simulink model "Stromregelkreis_old"  (R2024b)
settings: Solver=FixedStepAuto  StartTime=0.0  StopTime=inf  FixedStep=ta  RelTol=1e-3
PostLoadFcn:
  | if any(exist('dsrtsu_mdlpostloadfcn', 'file') ~= 0), dsrtsu_mdlpostloadfcn('Execute', bdroot); end
InitFcn:
  | , if any(exist('rtifpga_mdlclblib', 'file') ~= 0), rtifpga_mdlclblib('Init', bdroot); end,
undefined symbols (not defined in the file or in its folder): ta
libraries: rtilib1104 x20, simulink x4
settings Model: DSRTSU_INTERNAL_RTI_VER=650  DSRTSU_INTERNAL_RTI_TYPE=rti1104  DSRTSU_INTERNAL_RTIFPGA=210  DSRTSU_INTERNAL_RTISTBM_VER=24.2  Creator=115145  LastModifiedBy=217836
settings OptimizationCC: BlockReduction=off  OptimizeBlockIOStorage=off
settings HardwareCC: ProdBitPerPointer=32  ProdBitPerSizeT=32  ProdBitPerPtrDiffT=32  ProdLargestAtomicInteger=Integer  ProdEndianess=BigEndian  ProdWordSize=32  ProdHWDeviceType=Custom Processor->Custom  TargetIntDivRoundTo=Zero  TargetEndianess=BigEndian  TargetHWDeviceType=Custom Processor->Custom
settings SFSimCC: MATLABDynamicMemAlloc=off
settings RTWCC: Description=dSPACE DS1104 Hardware Platform  SystemTargetFile=rti1104.tlc  MakeCommand=make_rti  TemplateMakefile=rti1104.tmf
settings STFCustomTargetCC: ParMdlRefBuildCompliant=on  SystemTargetFile=rti1104.tlc
settings GRTTargetCC: TargetLangStandard=C89/C90 (ANSI)  CompOptLevelCompliant=off  ConcurrentExecutionCompliant=off  CombineOutputUpdateFcns=off  MatFileLogging=off  CPPClassGenCompliant=off  UseToolchainInfoCompliant=off

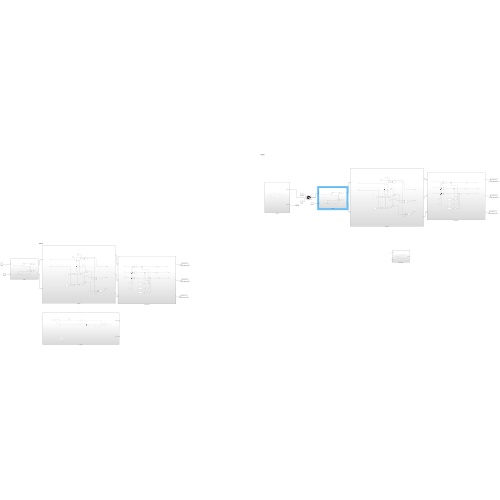
[thumbnail: Simulink's stored preview of the top-level diagram]
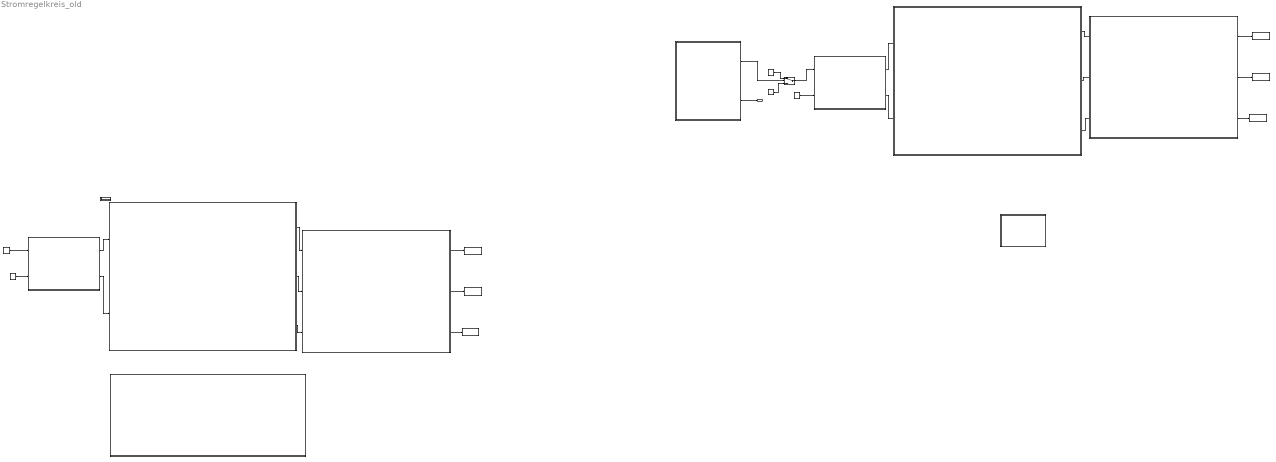
== system Stromregelkreis_old ==
  DS1104SL_DSP_BIT_OUT_C1 : rtilib1104/DS1104 SLAVE DSP/DS1104SL_DSP_BIT_OUT_C0  ChannelNo=1  InitValue=0  TermMode=0  TermValue=0  Reserved1=[]  Reserved2=[]  Reserved3=[]  Reserved=[]  DialogFcn=gui1104sl_dsp_bit_out  UnitName={'DS1104SL_DSP_BIT_OUT_C'}  UnitValues={1}  DSProperties=struct('RTI',struct('Version',uint32(1),'BlockType',struct('isSLSource',uint8(0),'isSLSink',uint8(1),'isHWSource',uint8(0),'isHWSink',uint8(1),'isSetup',uint8(0),'isInline',uint8(1),'isNonInline',uint8(0),'isInterrupt',uint8(0),'isChannelwise',uint8(1)),'IOBoardType','DS1104SLAVE','UnitType','BIT','Identifier','BITOUTCH','DialogType','ML','BlockSet','NONE','SlaveProcessor','F240'))
      settings: SourceProductName=dSPACE RTI1104
  DS1104SL_DSP_BIT_OUT_C2 : rtilib1104/DS1104 SLAVE DSP/DS1104SL_DSP_BIT_OUT_C0  ChannelNo=2  InitValue=0  TermMode=0  TermValue=0  Reserved1=[]  Reserved2=[]  Reserved3=[]  Reserved=[]  DialogFcn=gui1104sl_dsp_bit_out  UnitName={'DS1104SL_DSP_BIT_OUT_C'}  UnitValues={2}  DSProperties=struct('RTI',struct('Version',uint32(1),'BlockType',struct('isSLSource',uint8(0),'isSLSink',uint8(1),'isHWSource',uint8(0),'isHWSink',uint8(1),'isSetup',uint8(0),'isInline',uint8(1),'isNonInline',uint8(0),'isInterrupt',uint8(0),'isChannelwise',uint8(1)),'IOBoardType','DS1104SLAVE','UnitType','BIT','Identifier','BITOUTCH','DialogType','ML','BlockSet','NONE','SlaveProcessor','F240'))
      settings: SourceProductName=dSPACE RTI1104
  DS1104SL_DSP_BIT_OUT_C3 : rtilib1104/DS1104 SLAVE DSP/DS1104SL_DSP_BIT_OUT_C0  ChannelNo=3  InitValue=0  TermMode=0  TermValue=0  Reserved1=[]  Reserved2=[]  Reserved3=[]  Reserved=[]  DialogFcn=gui1104sl_dsp_bit_out  UnitName={'DS1104SL_DSP_BIT_OUT_C'}  UnitValues={ 3 }  DSProperties=struct('RTI',struct('Version',uint32(1),'BlockType',struct('isSLSource',uint8(0),'isSLSink',uint8(1),'isHWSource',uint8(0),'isHWSink',uint8(1),'isSetup',uint8(0),'isInline',uint8(1),'isNonInline',uint8(0),'isInterrupt',uint8(0),'isChannelwise',uint8(1)),'IOBoardType','DS1104SLAVE','UnitType','BIT','Identifier','BITOUTCH','DialogType','ML','BlockSet','NONE','SlaveProcessor','F240'))
      settings: SourceProductName=dSPACE RTI1104
  DS1104SL_DSP_BIT_OUT_C4 : rtilib1104/DS1104 SLAVE DSP/DS1104SL_DSP_BIT_OUT_C0  ChannelNo=4  InitValue=0  TermMode=0  TermValue=0  Reserved1=[]  Reserved2=[]  Reserved3=[]  Reserved=[]  DialogFcn=gui1104sl_dsp_bit_out  UnitName={'DS1104SL_DSP_BIT_OUT_C'}  UnitValues={ 4 }  DSProperties=struct('RTI',struct('Version',uint32(1),'BlockType',struct('isSLSource',uint8(0),'isSLSink',uint8(1),'isHWSource',uint8(0),'isHWSink',uint8(1),'isSetup',uint8(0),'isInline',uint8(1),'isNonInline',uint8(0),'isInterrupt',uint8(0),'isChannelwise',uint8(1)),'IOBoardType','DS1104SLAVE','UnitType','BIT','Identifier','BITOUTCH','DialogType','ML','BlockSet','NONE','SlaveProcessor','F240'))
      settings: SourceProductName=dSPACE RTI1104
  DS1104SL_DSP_BIT_OUT_C5 : rtilib1104/DS1104 SLAVE DSP/DS1104SL_DSP_BIT_OUT_C0  ChannelNo=5  InitValue=0  TermMode=0  TermValue=0  Reserved1=[]  Reserved2=[]  Reserved3=[]  Reserved=[]  DialogFcn=gui1104sl_dsp_bit_out  UnitName={'DS1104SL_DSP_BIT_OUT_C'}  UnitValues={ 5 }  DSProperties=struct('RTI',struct('Version',uint32(1),'BlockType',struct('isSLSource',uint8(0),'isSLSink',uint8(1),'isHWSource',uint8(0),'isHWSink',uint8(1),'isSetup',uint8(0),'isInline',uint8(1),'isNonInline',uint8(0),'isInterrupt',uint8(0),'isChannelwise',uint8(1)),'IOBoardType','DS1104SLAVE','UnitType','BIT','Identifier','BITOUTCH','DialogType','ML','BlockSet','NONE','SlaveProcessor','F240'))
      settings: SourceProductName=dSPACE RTI1104
  DS1104SL_DSP_BIT_OUT_C6 : rtilib1104/DS1104 SLAVE DSP/DS1104SL_DSP_BIT_OUT_C0  ChannelNo=6  InitValue=0  TermMode=0  TermValue=0  Reserved1=[]  Reserved2=[]  Reserved3=[]  Reserved=[]  DialogFcn=gui1104sl_dsp_bit_out  UnitName={'DS1104SL_DSP_BIT_OUT_C'}  UnitValues={6}  DSProperties=struct('RTI',struct('Version',uint32(1),'BlockType',struct('isSLSource',uint8(0),'isSLSink',uint8(1),'isHWSource',uint8(0),'isHWSink',uint8(1),'isSetup',uint8(0),'isInline',uint8(1),'isNonInline',uint8(0),'isInterrupt',uint8(0),'isChannelwise',uint8(1)),'IOBoardType','DS1104SLAVE','UnitType','BIT','Identifier','BITOUTCH','DialogType','ML','BlockSet','NONE','SlaveProcessor','F240'))
      settings: SourceProductName=dSPACE RTI1104
  Iq_soll : Constant  Value=0
  RTI Data : Subsystem  Tag=struct('RTIDataServer',struct('RTIDataServerVs','2','RTIModelDescription','struct(''main'',''Stromregelkreis_old'',''sub'',''Stromregelkreis_old'',''isMp'',0)'))  LoadFcn="if exist('rtidc'), try,  rtidc('DataHostBlockClbLoad', gcbh); catch, disp(['Warning: ''LoadFcn'' for RTI Data block failed: ' lasterr]); end, end,"  mask(RTI_DATA_HOST){}
      mask help:
      | RTI Data Block.
      | This block is used by RTI to store internal model-dependent data.
      | Please keep this block on the root level of the model. Deleting this block will result in data loss.
      |
      | NEVER DELETE OR COPY THIS BLOCK!
      settings: CopyFcn="if exist('rtidc'), try,  rtidc('DataHostBlockClbCopy', gcbh); catch, disp(['Warning: ''CopyFcn'' for RTI Data block failed: ' lasterr]); end, end,"  DeleteFcn="if exist('rtidc'), try,  rtidc('DataHostBlockClbDelete', gcbh); catch, disp(['Warning: ''DeleteFcn'' for RTI Data block failed: ' lasterr]); end, end,"  ModelCloseFcn="if exist('rtidc'), try,  rtidc('DataHostBlockClbModelClose', gcbh); catch, disp(['Warning: ''ModelCloseFcn'' for RTI Data block failed: ' lasterr]); end, end,"  PreSaveFcn="if exist('rtidc'), try,  rtidc('DataHostBlockClbPreSave', gcbh); catch, disp(['Warning: ''PreSaveFcn'' for RTI Data block failed: ' lasterr]); end, end,"  PostSaveFcn="if exist('rtidc'), try,  rtidc('DataHostBlockClbPostSave', gcbh); catch, disp(['Warning: ''PostSaveFcn'' for RTI Data block failed: ' lasterr]); end, end,"  NameChangeFcn="if exist('rtidc'), try,  rtidc('DataHostBlockClbNameChange', gcbh); catch, disp(['Warning: ''NameChangeFcn'' for RTI Data block failed: ' lasterr]); end, end,"
      mask Help:
      | RTI Data Block.
      | This block is used by RTI to store internal model-dependent data.
      | Please keep this block on the root level of the model. Deleting this block will result in data loss.
      | 
      | NEVER DELETE OR COPY THIS BLOCK!
      mask Display:
      | text(0.5, 0.5, 'RTI Data', 'HorizontalAlignment', 'center');
      | plot([1 0]);
  Ramp : simulink/Sources/Ramp  slope=6*pi  start=0  InitialOutput=0
  Ramp1 : simulink/Sources/Ramp  slope=6*pi  start=0  InitialOutput=0
  Stromregelung : Subsystem
  Stromregelung1 : Subsystem
  dq>ab : Subsystem
  dq>ab1 : Subsystem
  drehzahlregler1 : Subsystem
  encoder : Subsystem
  encoder1 : Subsystem
  iq_soll : Constant  Value=0
  iq_soll_enable_sw : Switch  SaturateOnIntegerOverflow=off  InputSameDT=off
  iq_soll_safe : Constant  Value=0
  lageregler : Subsystem
  lageregler1 : Subsystem
  Ist_Drehzahl : Outport
  wires:
  Stromregelung/1(Out1) -> DS1104SL_DSP_BIT_OUT_C3/1
  Stromregelung/2(Out2) -> DS1104SL_DSP_BIT_OUT_C4/1
  Stromregelung/3(Out3) -> DS1104SL_DSP_BIT_OUT_C5/1
  Iq_soll/1 -> dq>ab/1(In1)
  Ramp/1 -> dq>ab/2(In2)
  dq>ab/1(Out1) -> lageregler/1(In2)
  dq>ab/2(Out2) -> lageregler/2(In3)
  lageregler/1(Out1) -> Stromregelung/1(In1)
  lageregler/2(Out2) -> Stromregelung/2(In2)
  lageregler/3(Out3) -> Stromregelung/3(In3)
  encoder1/2(Ist_Drehzahl) -> Ist_Drehzahl/1
  iq_soll/1 -> iq_soll_enable_sw/3
  Stromregelung1/2(Out2) -> DS1104SL_DSP_BIT_OUT_C2/1
  encoder1/1(gamma_ref) -> iq_soll_enable_sw/2
  iq_soll_enable_sw/1 -> dq>ab1/1(In1)  "iq_soll_final"
  lageregler1/2(Out2) -> Stromregelung1/2(In2)
  iq_soll_safe/1 -> iq_soll_enable_sw/1
  lageregler1/1(Out1) -> Stromregelung1/1(In1)
  Stromregelung1/1(Out1) -> DS1104SL_DSP_BIT_OUT_C1/1
  lageregler1/3(Out3) -> Stromregelung1/3(In3)
  dq>ab1/2(Out2) -> lageregler1/2(In3)
  Stromregelung1/3(Out3) -> DS1104SL_DSP_BIT_OUT_C6/1
  dq>ab1/1(Out1) -> lageregler1/1(In2)
  Ramp1/1 -> dq>ab1/2(In2)

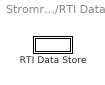
== system Stromregelkreis_old/RTI Data ==
  RTI Data Store : Subsystem  Tag="struct('private',struct('version',struct('dsVer',uint32(2),'dsVerCreation',uint32(2),'RTI',struct('ver','24.2','type','RTI1104')),'access',struct('type','Model','isPerm',1,'created',['13-Jan-2026 19:21:42'],'location','')),'public',struct('main',struct('data',[]),'sub',struct('name',{{'Stromregelkreis_old'}},'data',{{struct('TH',struct('thTaskInfo',struct('taskType',{'TIMER','HWINT','TMRINT','SWINT','GLINT'},'tasksNumOf',{1,0,0,0,0},'srcIds',{{'TIMERA'},{},{},{},{}},'taskNames',{{['Timer Task 1']},{},{},{},{}})),'th_tc',struct('dataType','TASK','taskGroupId','','taskGroupList',{{}},'taskSchedulingPolicy','FCFS','taskType','TIMER','blkh',-1,'srcId','TIMERA','srcSgnName',['Timer A interrupt'],'srcCpuName','','taskName',['Timer Task 1  [5e-05] s'],'taskNameDisplayExt','','smplTime',5e-5,'smplTimeOffs',0,'hasFixedPriority',0,'priority',1,'hasFixedOvc',0,'ovcType',1,'ovcMax',1),'tc_th',struct('dataType','TASK','taskGroupId','','taskGroupList',{{}},'taskSchedulingPolicy','FCFS','taskType','TIMER','blkh',-1,'srcId','TIMERA','srcSgnName',['Timer A interrupt'],'srcCpuName','','taskName',['Timer Task 1  [5e-05] s'],'taskNameDisplayExt','','smplTime',5e-5,'smplTimeOffs',0,'hasFixedPriority',0,'priority',1,'hasFixedOvc',0,'ovcType',1,'ovcMax',1))}})))"  mask(RTI_DATA_STORE){}
      mask help:
      | RTI Data Store Block. This block is used by RTI to store internal model dependent data. Deleting this block will result in data loss.
      |
      | NEVER DELETE, COPY, OR MODIFY THIS BLOCK!
      mask Help:
      | RTI Data Store Block. This block is used by RTI to store internal model dependent data. Deleting this block will result in data loss.
      | 
      | NEVER DELETE, COPY, OR MODIFY THIS BLOCK!
      mask Display: text(0.5, 0.5, ' ', 'HorizontalAlignment', 'center');

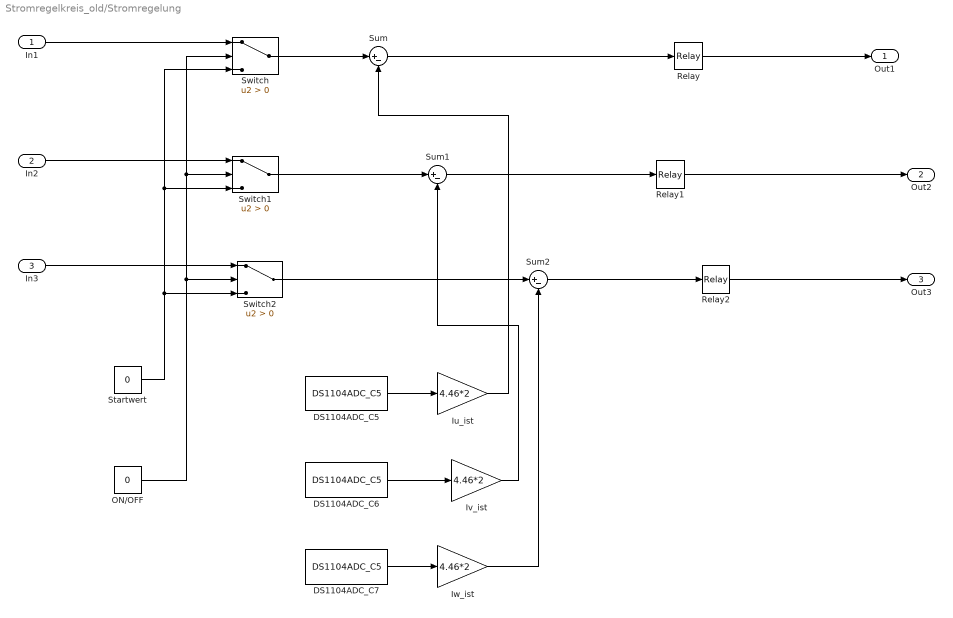
== system Stromregelkreis_old/Stromregelung ==
  In1 : Inport
  In2 : Inport  Port=2
  In3 : Inport  Port=3
  DS1104ADC_C5 : rtilib1104/DS1104 MASTER PPC/DS1104ADC_C5  ChannelNo=5  TriggerMode=0  Reserved1=[]  Reserved2=[]  Reserved3=[]  Reserved4=[]  DialogFcn=gui1104adc  UnitName={ 'DS1104ADC_C' }  UnitValues={ 5 }  DSProperties=struct('RTI',struct('Version',uint32(1),'BlockType',struct('isSLSource',uint8(1),'isSLSink',uint8(0),'isHWSource',uint8(1),'isHWSink',uint8(0),'isSetup',uint8(0),'isInline',uint8(1),'isNonInline',uint8(0),'isInterrupt',uint8(0),'isChannelwise',uint8(1)),'IOBoardType','DS1104MASTER','UnitType','ADC','Identifier','ADC','DialogType','ML','BlockSet','NONE','SlaveProcessor','NONE'))
      settings: SourceProductName=dSPACE RTI1104
  DS1104ADC_C6 : rtilib1104/DS1104 MASTER PPC/DS1104ADC_C5  ChannelNo=6  TriggerMode=0  Reserved1=[]  Reserved2=[]  Reserved3=[]  Reserved4=[]  DialogFcn=gui1104adc  UnitName={ 'DS1104ADC_C' }  UnitValues={ 6 }  DSProperties=struct('RTI',struct('Version',uint32(1),'BlockType',struct('isSLSource',uint8(1),'isSLSink',uint8(0),'isHWSource',uint8(1),'isHWSink',uint8(0),'isSetup',uint8(0),'isInline',uint8(1),'isNonInline',uint8(0),'isInterrupt',uint8(0),'isChannelwise',uint8(1)),'IOBoardType','DS1104MASTER','UnitType','ADC','Identifier','ADC','DialogType','ML','BlockSet','NONE','SlaveProcessor','NONE'))
      settings: SourceProductName=dSPACE RTI1104
  DS1104ADC_C7 : rtilib1104/DS1104 MASTER PPC/DS1104ADC_C5  ChannelNo=7  TriggerMode=0  Reserved1=[]  Reserved2=[]  Reserved3=[]  Reserved4=[]  DialogFcn=gui1104adc  UnitName={ 'DS1104ADC_C' }  UnitValues={ 7 }  DSProperties=struct('RTI',struct('Version',uint32(1),'BlockType',struct('isSLSource',uint8(1),'isSLSink',uint8(0),'isHWSource',uint8(1),'isHWSink',uint8(0),'isSetup',uint8(0),'isInline',uint8(1),'isNonInline',uint8(0),'isInterrupt',uint8(0),'isChannelwise',uint8(1)),'IOBoardType','DS1104MASTER','UnitType','ADC','Identifier','ADC','DialogType','ML','BlockSet','NONE','SlaveProcessor','NONE'))
      settings: SourceProductName=dSPACE RTI1104
  Iu_ist : Gain  Gain=4.46*2
  Iv_ist : Gain  Gain=4.46*2
  Iw_ist : Gain  Gain=4.46*2
  ON/OFF : Constant  Value=0
  Relay : Relay  OnSwitchValue=0.1  OffSwitchValue=-0.1  OutDataTypeStr=Inherit: Inherit via back propagation
  Relay1 : Relay  OnSwitchValue=0.1  OffSwitchValue=-0.1  OutDataTypeStr=Inherit: Inherit via back propagation
  Relay2 : Relay  OnSwitchValue=0.1  OffSwitchValue=-0.1  OutDataTypeStr=Inherit: Inherit via back propagation
  Startwert : Constant  Value=0
  Sum : Sum  Inputs=|+-
  Sum1 : Sum  Inputs=|+-
  Sum2 : Sum  Inputs=|+-
  Switch : Switch  Criteria=u2 > Threshold  SaturateOnIntegerOverflow=off  InputSameDT=off
  Switch1 : Switch  Criteria=u2 > Threshold  SaturateOnIntegerOverflow=off  InputSameDT=off
  Switch2 : Switch  Criteria=u2 > Threshold  SaturateOnIntegerOverflow=off  InputSameDT=off
  Out1 : Outport
  Out2 : Outport  Port=2
  Out3 : Outport  Port=3
  wires:
  DS1104ADC_C7/1 -> Iw_ist/1
  Sum2/1 -> Relay2/1
  In2/1 -> Switch1/1
  ON/OFF/1 -> Switch1/2, Switch/2, Switch2/2
  Startwert/1 -> Switch2/3, Switch/3, Switch1/3
  In1/1 -> Switch/1
  Iu_ist/1 -> Sum/2
  Switch/1 -> Sum/1
  DS1104ADC_C5/1 -> Iu_ist/1
  Switch2/1 -> Sum2/1
  Sum1/1 -> Relay1/1
  Sum/1 -> Relay/1
  Iv_ist/1 -> Sum1/2
  Iw_ist/1 -> Sum2/2
  DS1104ADC_C6/1 -> Iv_ist/1
  Switch1/1 -> Sum1/1
  Relay2/1 -> Out3/1
  Relay/1 -> Out1/1
  Relay1/1 -> Out2/1
  In3/1 -> Switch2/1

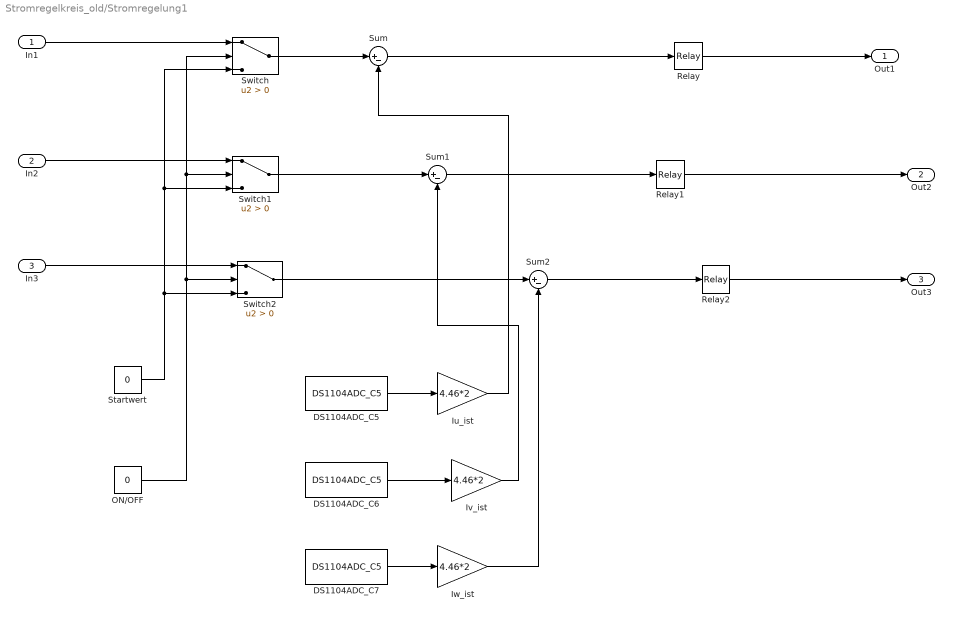
== system Stromregelkreis_old/Stromregelung1 ==
  In1 : Inport
  In2 : Inport  Port=2
  In3 : Inport  Port=3
  DS1104ADC_C5 : rtilib1104/DS1104 MASTER PPC/DS1104ADC_C5  ChannelNo=5  TriggerMode=0  Reserved1=[]  Reserved2=[]  Reserved3=[]  Reserved4=[]  DialogFcn=gui1104adc  UnitName={ 'DS1104ADC_C' }  UnitValues={ 5 }  DSProperties=struct('RTI',struct('Version',uint32(1),'BlockType',struct('isSLSource',uint8(1),'isSLSink',uint8(0),'isHWSource',uint8(1),'isHWSink',uint8(0),'isSetup',uint8(0),'isInline',uint8(1),'isNonInline',uint8(0),'isInterrupt',uint8(0),'isChannelwise',uint8(1)),'IOBoardType','DS1104MASTER','UnitType','ADC','Identifier','ADC','DialogType','ML','BlockSet','NONE','SlaveProcessor','NONE'))
      settings: SourceProductName=dSPACE RTI1104
  DS1104ADC_C6 : rtilib1104/DS1104 MASTER PPC/DS1104ADC_C5  ChannelNo=6  TriggerMode=0  Reserved1=[]  Reserved2=[]  Reserved3=[]  Reserved4=[]  DialogFcn=gui1104adc  UnitName={ 'DS1104ADC_C' }  UnitValues={ 6 }  DSProperties=struct('RTI',struct('Version',uint32(1),'BlockType',struct('isSLSource',uint8(1),'isSLSink',uint8(0),'isHWSource',uint8(1),'isHWSink',uint8(0),'isSetup',uint8(0),'isInline',uint8(1),'isNonInline',uint8(0),'isInterrupt',uint8(0),'isChannelwise',uint8(1)),'IOBoardType','DS1104MASTER','UnitType','ADC','Identifier','ADC','DialogType','ML','BlockSet','NONE','SlaveProcessor','NONE'))
      settings: SourceProductName=dSPACE RTI1104
  DS1104ADC_C7 : rtilib1104/DS1104 MASTER PPC/DS1104ADC_C5  ChannelNo=7  TriggerMode=0  Reserved1=[]  Reserved2=[]  Reserved3=[]  Reserved4=[]  DialogFcn=gui1104adc  UnitName={ 'DS1104ADC_C' }  UnitValues={ 7 }  DSProperties=struct('RTI',struct('Version',uint32(1),'BlockType',struct('isSLSource',uint8(1),'isSLSink',uint8(0),'isHWSource',uint8(1),'isHWSink',uint8(0),'isSetup',uint8(0),'isInline',uint8(1),'isNonInline',uint8(0),'isInterrupt',uint8(0),'isChannelwise',uint8(1)),'IOBoardType','DS1104MASTER','UnitType','ADC','Identifier','ADC','DialogType','ML','BlockSet','NONE','SlaveProcessor','NONE'))
      settings: SourceProductName=dSPACE RTI1104
  Iu_ist : Gain  Gain=4.46*2
  Iv_ist : Gain  Gain=4.46*2
  Iw_ist : Gain  Gain=4.46*2
  ON/OFF : Constant  Value=0
  Relay : Relay  OnSwitchValue=0.1  OffSwitchValue=-0.1  OutDataTypeStr=Inherit: Inherit via back propagation
  Relay1 : Relay  OnSwitchValue=0.1  OffSwitchValue=-0.1  OutDataTypeStr=Inherit: Inherit via back propagation
  Relay2 : Relay  OnSwitchValue=0.1  OffSwitchValue=-0.1  OutDataTypeStr=Inherit: Inherit via back propagation
  Startwert : Constant  Value=0
  Sum : Sum  Inputs=|+-
  Sum1 : Sum  Inputs=|+-
  Sum2 : Sum  Inputs=|+-
  Switch : Switch  Criteria=u2 > Threshold  SaturateOnIntegerOverflow=off  InputSameDT=off
  Switch1 : Switch  Criteria=u2 > Threshold  SaturateOnIntegerOverflow=off  InputSameDT=off
  Switch2 : Switch  Criteria=u2 > Threshold  SaturateOnIntegerOverflow=off  InputSameDT=off
  Out1 : Outport
  Out2 : Outport  Port=2
  Out3 : Outport  Port=3
  wires:
  DS1104ADC_C7/1 -> Iw_ist/1
  Sum2/1 -> Relay2/1
  In2/1 -> Switch1/1
  ON/OFF/1 -> Switch1/2, Switch/2, Switch2/2
  Startwert/1 -> Switch2/3, Switch/3, Switch1/3
  In1/1 -> Switch/1
  Iu_ist/1 -> Sum/2
  Switch/1 -> Sum/1
  DS1104ADC_C5/1 -> Iu_ist/1
  Switch2/1 -> Sum2/1
  Sum1/1 -> Relay1/1
  Sum/1 -> Relay/1
  Iv_ist/1 -> Sum1/2
  Iw_ist/1 -> Sum2/2
  DS1104ADC_C6/1 -> Iv_ist/1
  Switch1/1 -> Sum1/1
  Relay2/1 -> Out3/1
  Relay/1 -> Out1/1
  Relay1/1 -> Out2/1
  In3/1 -> Switch2/1

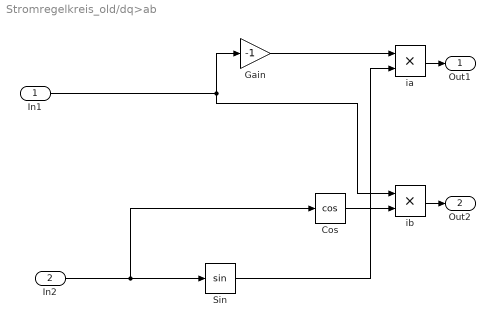
== system Stromregelkreis_old/dq>ab ==
  In1 : Inport
  In2 : Inport  Port=2
  Cos : Trigonometry  Operator=cos
  Gain : Gain  Gain=-1
  Sin : Trigonometry
  ia : Product
  ib : Product
  Out1 : Outport
  Out2 : Outport  Port=2
  wires:
  In2/1 -> Cos/1, Sin/1
  ia/1 -> Out1/1
  In1/1 -> ib/1, Gain/1
  Gain/1 -> ia/1
  Cos/1 -> ib/2
  Sin/1 -> ia/2
  ib/1 -> Out2/1

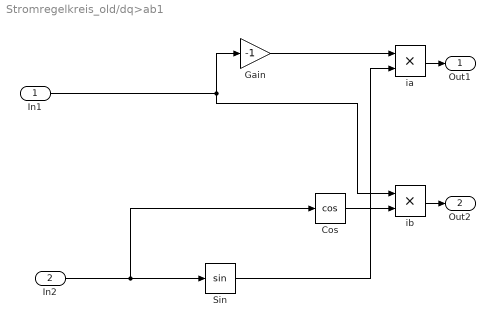
== system Stromregelkreis_old/dq>ab1 ==
  In1 : Inport
  In2 : Inport  Port=2
  Cos : Trigonometry  Operator=cos
  Gain : Gain  Gain=-1
  Sin : Trigonometry
  ia : Product
  ib : Product
  Out1 : Outport
  Out2 : Outport  Port=2
  wires:
  In2/1 -> Cos/1, Sin/1
  ia/1 -> Out1/1
  In1/1 -> ib/1, Gain/1
  Gain/1 -> ia/1
  Cos/1 -> ib/2
  Sin/1 -> ia/2
  ib/1 -> Out2/1

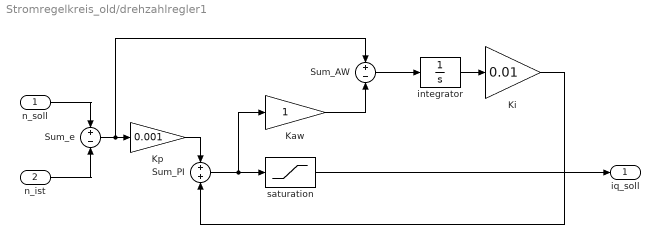
== system Stromregelkreis_old/drehzahlregler1 ==
  n_soll : Inport
  n_ist : Inport  Port=2
  Kaw : Gain
  Ki : Gain  Gain=0.01
  Kp : Gain  Gain=0.001
  Sum_AW : Sum  Inputs=+-
  Sum_PI : Sum
  Sum_e : Sum  Inputs=+-
  integrator : Integrator
  saturation : Saturate  UpperLimit=1  LowerLimit=-1
  iq_soll : Outport
  wires:
  n_soll/1 -> Sum_e/1
  Sum_PI/1 -> saturation/1, Kaw/1
  Kp/1 -> Sum_PI/1
  n_ist/1 -> Sum_e/2
  Sum_e/1 -> Sum_AW/1, Kp/1
  Sum_AW/1 -> integrator/1
  saturation/1 -> iq_soll/1
  Kaw/1 -> Sum_AW/2
  integrator/1 -> Ki/1
  Ki/1 -> Sum_PI/2

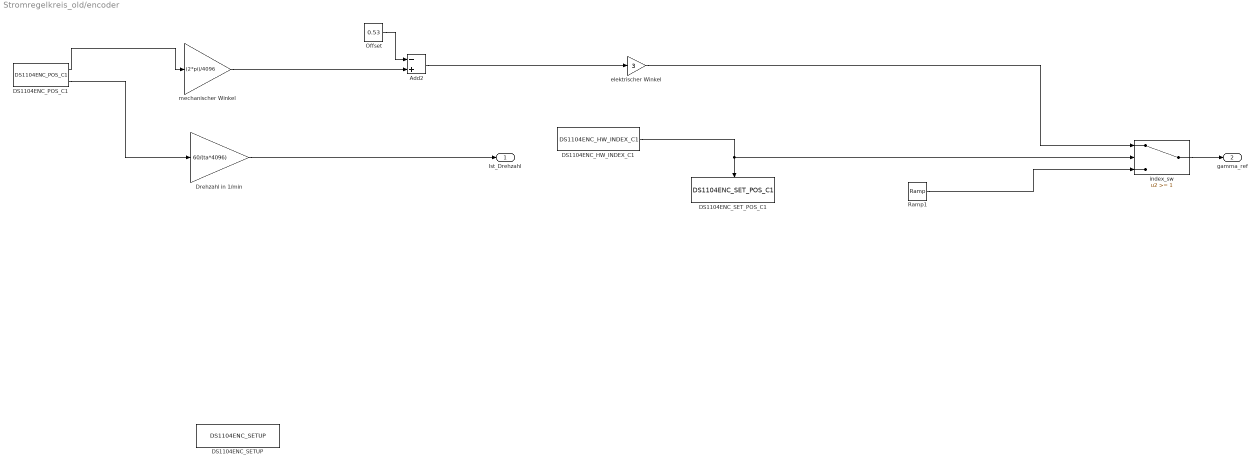
== system Stromregelkreis_old/encoder ==
  Add2 : Sum  Inputs=-+
  DS1104ENC_HW_INDEX_C1 : rtilib1104/DS1104 MASTER PPC/DS1104ENC_HW_INDEX_C1  ChannelNo=1  SetPosMode=2  SetOutMode=1  Reserved1=[]  Reserved2=[]  Reserved3=[]  Reserved4=[]  DialogFcn=gui1104enc_hw_index  UnitName={'DS1104ENC_HW_INDEX_C'}  UnitValues={ 1 }  DSProperties=struct('RTI',struct('Version',uint32(1),'BlockType',struct('isSLSource',uint8(1),'isSLSink',uint8(0),'isHWSource',uint8(1),'isHWSink',uint8(0),'isSetup',uint8(0),'isInline',uint8(1),'isNonInline',uint8(0),'isInterrupt',uint8(0),'isChannelwise',uint8(1)),'IOBoardType','DS1104MASTER','UnitType','ENC','Identifier','ENCINDEXHW','DialogType','ML','BlockSet','NONE','SlaveProcessor','NONE'))
      settings: SourceProductName=dSPACE RTI1104
  DS1104ENC_POS_C1 : rtilib1104/DS1104 MASTER PPC/DS1104ENC_POS_C1  ChannelNo=1  PosValue=0  Reserved1=[]  Reserved2=[]  Reserved3=[]  Reserved4=[]  DialogFcn=gui1104enc_pos  UnitName={'DS1104ENC_POS_C'}  UnitValues={ 1 }  DSProperties=struct('RTI',struct('Version',uint32(1),'BlockType',struct('isSLSource',uint8(1),'isSLSink',uint8(0),'isHWSource',uint8(1),'isHWSink',uint8(0),'isSetup',uint8(0),'isInline',uint8(1),'isNonInline',uint8(0),'isInterrupt',uint8(0),'isChannelwise',uint8(1)),'IOBoardType','DS1104MASTER','UnitType','ENC','Identifier','ENCPOSCH','DialogType','ML','BlockSet','NONE','SlaveProcessor','NONE'))
      settings: SourceProductName=dSPACE RTI1104
  DS1104ENC_SETUP : rtilib1104/DS1104 MASTER PPC/DS1104ENC_SETUP  Reserved1=[]  Reserved2=[]  Reserved3=[]  Reserved4=[]  DialogFcn=gui1104enc_setup  UnitName={'DS1104ENC_SETUP'}  UnitValues={ [] }  DSProperties=struct('RTI',struct('Version',uint32(1),'BlockType',struct('isSLSource',uint8(0),'isSLSink',uint8(0),'isHWSource',uint8(0),'isHWSink',uint8(0),'isSetup',uint8(0),'isInline',uint8(1),'isNonInline',uint8(0),'isInterrupt',uint8(0),'isChannelwise',uint8(0)),'IOBoardType','DS1104MASTER','UnitType','ENC','Identifier','ENCSETUP','DialogType','ML','BlockSet','NONE','SlaveProcessor','NONE'))
      settings: SourceProductName=dSPACE RTI1104  SignalType=[0 0]
  DS1104ENC_SET_POS_C1 : rtilib1104/DS1104 MASTER PPC/DS1104ENC_SET_POS_C1  ChannelNo=1  PosValue=0  Reserved1=[]  Reserved2=[]  Reserved3=[]  Reserved4=[]  DialogFcn=gui1104enc_set_pos  UnitName={'DS1104ENC_SET_POS_C'}  UnitValues={ 1 }  DSProperties=struct('RTI',struct('Version',uint32(1),'BlockType',struct('isSLSource',uint8(0),'isSLSink',uint8(1),'isHWSource',uint8(0),'isHWSink',uint8(1),'isSetup',uint8(0),'isInline',uint8(1),'isNonInline',uint8(0),'isInterrupt',uint8(0),'isChannelwise',uint8(1)),'IOBoardType','DS1104MASTER','UnitType','ENC','Identifier','ENCRESET','DialogType','ML','BlockSet','NONE','SlaveProcessor','NONE'))
      settings: SourceProductName=dSPACE RTI1104
  Drehzahl in 1/min : Gain  Gain=60/(ta*4096)
  Offset : Constant  Value=0.53
  Ramp1 : simulink/Sources/Ramp  slope=6*pi  start=0  InitialOutput=0
  elektrischer Winkel : Gain  Gain=3
  index_sw : Switch  Threshold=1  SaturateOnIntegerOverflow=off  InputSameDT=off
  mechanischer Winkel : Gain  Gain=(2*pi)/4096
  Ist_Drehzahl : Outport
  gamma_ref : Outport  Port=2
  wires:
  DS1104ENC_POS_C1/2 -> Drehzahl in 1/min/1
  DS1104ENC_POS_C1/1 -> mechanischer Winkel/1
  Add2/1 -> elektrischer Winkel/1
  mechanischer Winkel/1 -> Add2/2
  Offset/1 -> Add2/1
  Drehzahl in 1/min/1 -> Ist_Drehzahl/1
  DS1104ENC_HW_INDEX_C1/1 -> index_sw/2, DS1104ENC_SET_POS_C1/Trigger
  elektrischer Winkel/1 -> index_sw/1
  index_sw/1 -> gamma_ref/1
  Ramp1/1 -> index_sw/3

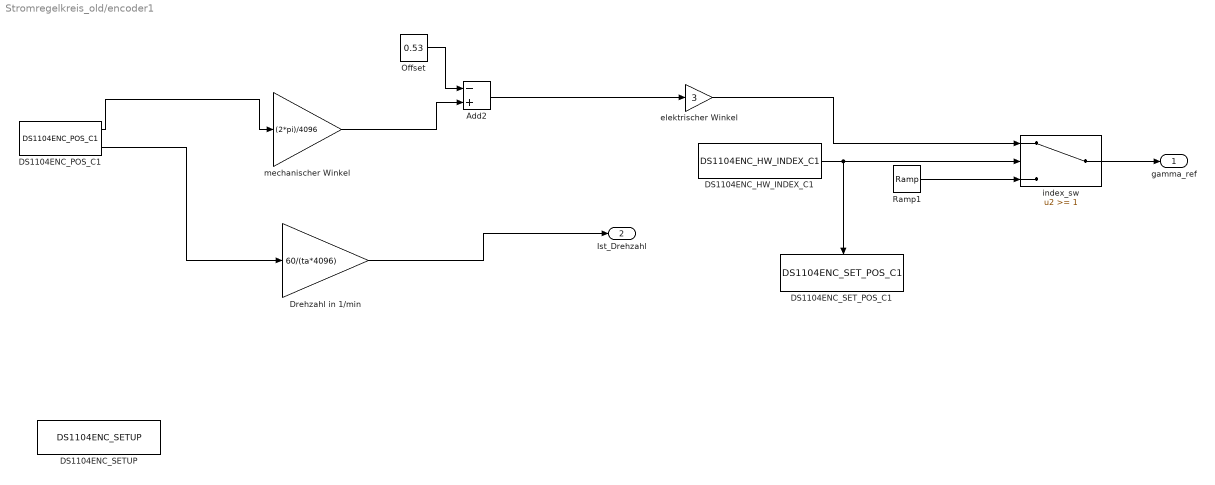
== system Stromregelkreis_old/encoder1 ==
  Add2 : Sum  Inputs=-+
  DS1104ENC_HW_INDEX_C1 : rtilib1104/DS1104 MASTER PPC/DS1104ENC_HW_INDEX_C1  ChannelNo=1  SetPosMode=2  SetOutMode=1  Reserved1=[]  Reserved2=[]  Reserved3=[]  Reserved4=[]  DialogFcn=gui1104enc_hw_index  UnitName={'DS1104ENC_HW_INDEX_C'}  UnitValues={ 1 }  DSProperties=struct('RTI',struct('Version',uint32(1),'BlockType',struct('isSLSource',uint8(1),'isSLSink',uint8(0),'isHWSource',uint8(1),'isHWSink',uint8(0),'isSetup',uint8(0),'isInline',uint8(1),'isNonInline',uint8(0),'isInterrupt',uint8(0),'isChannelwise',uint8(1)),'IOBoardType','DS1104MASTER','UnitType','ENC','Identifier','ENCINDEXHW','DialogType','ML','BlockSet','NONE','SlaveProcessor','NONE'))
      settings: SourceProductName=dSPACE RTI1104
  DS1104ENC_POS_C1 : rtilib1104/DS1104 MASTER PPC/DS1104ENC_POS_C1  ChannelNo=1  PosValue=0  Reserved1=[]  Reserved2=[]  Reserved3=[]  Reserved4=[]  DialogFcn=gui1104enc_pos  UnitName={'DS1104ENC_POS_C'}  UnitValues={ 1 }  DSProperties=struct('RTI',struct('Version',uint32(1),'BlockType',struct('isSLSource',uint8(1),'isSLSink',uint8(0),'isHWSource',uint8(1),'isHWSink',uint8(0),'isSetup',uint8(0),'isInline',uint8(1),'isNonInline',uint8(0),'isInterrupt',uint8(0),'isChannelwise',uint8(1)),'IOBoardType','DS1104MASTER','UnitType','ENC','Identifier','ENCPOSCH','DialogType','ML','BlockSet','NONE','SlaveProcessor','NONE'))
      settings: SourceProductName=dSPACE RTI1104
  DS1104ENC_SETUP : rtilib1104/DS1104 MASTER PPC/DS1104ENC_SETUP  Reserved1=[]  Reserved2=[]  Reserved3=[]  Reserved4=[]  DialogFcn=gui1104enc_setup  UnitName={'DS1104ENC_SETUP'}  UnitValues={ [] }  DSProperties=struct('RTI',struct('Version',uint32(1),'BlockType',struct('isSLSource',uint8(0),'isSLSink',uint8(0),'isHWSource',uint8(0),'isHWSink',uint8(0),'isSetup',uint8(0),'isInline',uint8(1),'isNonInline',uint8(0),'isInterrupt',uint8(0),'isChannelwise',uint8(0)),'IOBoardType','DS1104MASTER','UnitType','ENC','Identifier','ENCSETUP','DialogType','ML','BlockSet','NONE','SlaveProcessor','NONE'))
      settings: SourceProductName=dSPACE RTI1104  SignalType=[0 0]
  DS1104ENC_SET_POS_C1 : rtilib1104/DS1104 MASTER PPC/DS1104ENC_SET_POS_C1  ChannelNo=1  PosValue=0  Reserved1=[]  Reserved2=[]  Reserved3=[]  Reserved4=[]  DialogFcn=gui1104enc_set_pos  UnitName={'DS1104ENC_SET_POS_C'}  UnitValues={ 1 }  DSProperties=struct('RTI',struct('Version',uint32(1),'BlockType',struct('isSLSource',uint8(0),'isSLSink',uint8(1),'isHWSource',uint8(0),'isHWSink',uint8(1),'isSetup',uint8(0),'isInline',uint8(1),'isNonInline',uint8(0),'isInterrupt',uint8(0),'isChannelwise',uint8(1)),'IOBoardType','DS1104MASTER','UnitType','ENC','Identifier','ENCRESET','DialogType','ML','BlockSet','NONE','SlaveProcessor','NONE'))
      settings: SourceProductName=dSPACE RTI1104
  Drehzahl in 1/min : Gain  Gain=60/(ta*4096)
  Offset : Constant  Value=0.53
  Ramp1 : simulink/Sources/Ramp  slope=6*pi  start=0  InitialOutput=0
  elektrischer Winkel : Gain  Gain=3
  index_sw : Switch  Threshold=1  SaturateOnIntegerOverflow=off  InputSameDT=off
  mechanischer Winkel : Gain  Gain=(2*pi)/4096
  gamma_ref : Outport
  Ist_Drehzahl : Outport  Port=2
  wires:
  DS1104ENC_HW_INDEX_C1/1 -> DS1104ENC_SET_POS_C1/Trigger, index_sw/2
  index_sw/1 -> gamma_ref/1
  Ramp1/1 -> index_sw/3
  elektrischer Winkel/1 -> index_sw/1
  DS1104ENC_POS_C1/2 -> Drehzahl in 1/min/1
  DS1104ENC_POS_C1/1 -> mechanischer Winkel/1
  Add2/1 -> elektrischer Winkel/1
  Drehzahl in 1/min/1 -> Ist_Drehzahl/1
  Offset/1 -> Add2/1
  mechanischer Winkel/1 -> Add2/2

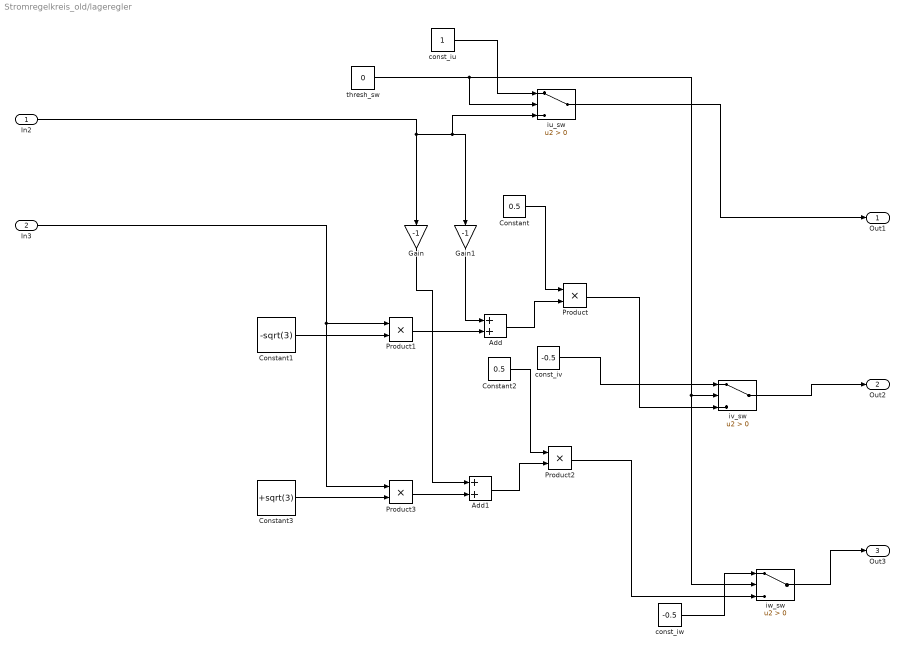
== system Stromregelkreis_old/lageregler ==
  In2 : Inport
  In3 : Inport  Port=2
  Add : Sum
  Add1 : Sum
  Constant : Constant  Value=0.5
  Constant1 : Constant  Value=-sqrt(3)
  Constant2 : Constant  Value=0.5
  Constant3 : Constant  Value=+sqrt(3)
  Gain : Gain  Gain=-1
  Gain1 : Gain  Gain=-1
  Product{,1..3} (4 alike) : Product
  const_iu : Constant
  const_iv : Constant  Value=-0.5
  const_iw : Constant  Value=-0.5
  iu_sw : Switch  Criteria=u2 > Threshold  SaturateOnIntegerOverflow=off  InputSameDT=off
  iv_sw : Switch  Criteria=u2 > Threshold  SaturateOnIntegerOverflow=off  InputSameDT=off
  iw_sw : Switch  Criteria=u2 > Threshold  SaturateOnIntegerOverflow=off  InputSameDT=off
  thresh_sw : Constant  Value=0
  Out1 : Outport
  Out2 : Outport  Port=2
  Out3 : Outport  Port=3
  wires:
  In3/1 -> Product3/1, Product1/1
  Add/1 -> Product/2
  Product1/1 -> Add/2
  In2/1 -> iu_sw/3, Gain1/1, Gain/1
  Constant/1 -> Product/1
  Product3/1 -> Add1/2
  Add1/1 -> Product2/2
  const_iu/1 -> iu_sw/1
  Constant1/1 -> Product1/2
  Constant3/1 -> Product3/2
  Gain/1 -> Add1/1
  iv_sw/1 -> Out2/1
  Gain1/1 -> Add/1
  Constant2/1 -> Product2/1
  iw_sw/1 -> Out3/1
  iu_sw/1 -> Out1/1
  thresh_sw/1 -> iw_sw/2, iv_sw/2, iu_sw/2
  Product/1 -> iv_sw/3
  const_iv/1 -> iv_sw/1
  Product2/1 -> iw_sw/3
  const_iw/1 -> iw_sw/1

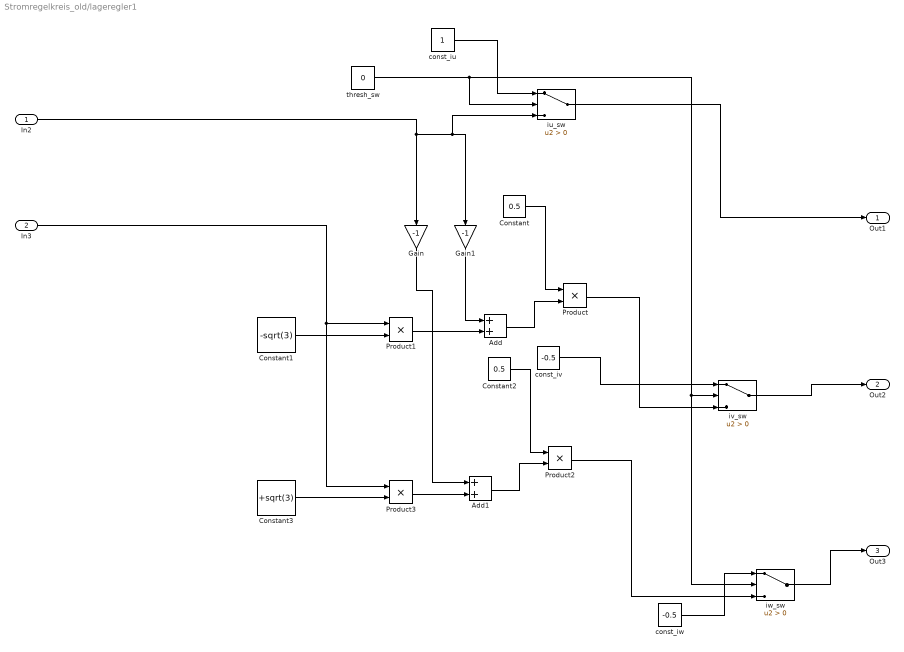
== system Stromregelkreis_old/lageregler1 ==
  In2 : Inport
  In3 : Inport  Port=2
  Add : Sum
  Add1 : Sum
  Constant : Constant  Value=0.5
  Constant1 : Constant  Value=-sqrt(3)
  Constant2 : Constant  Value=0.5
  Constant3 : Constant  Value=+sqrt(3)
  Gain : Gain  Gain=-1
  Gain1 : Gain  Gain=-1
  Product{,1..3} (4 alike) : Product
  const_iu : Constant
  const_iv : Constant  Value=-0.5
  const_iw : Constant  Value=-0.5
  iu_sw : Switch  Criteria=u2 > Threshold  SaturateOnIntegerOverflow=off  InputSameDT=off
  iv_sw : Switch  Criteria=u2 > Threshold  SaturateOnIntegerOverflow=off  InputSameDT=off
  iw_sw : Switch  Criteria=u2 > Threshold  SaturateOnIntegerOverflow=off  InputSameDT=off
  thresh_sw : Constant  Value=0
  Out1 : Outport
  Out2 : Outport  Port=2
  Out3 : Outport  Port=3
  wires:
  In3/1 -> Product3/1, Product1/1
  Add/1 -> Product/2
  Product1/1 -> Add/2
  In2/1 -> iu_sw/3, Gain1/1, Gain/1
  Constant/1 -> Product/1
  Product3/1 -> Add1/2
  Add1/1 -> Product2/2
  const_iu/1 -> iu_sw/1
  Constant1/1 -> Product1/2
  Constant3/1 -> Product3/2
  Gain/1 -> Add1/1
  iv_sw/1 -> Out2/1
  Gain1/1 -> Add/1
  Constant2/1 -> Product2/1
  iw_sw/1 -> Out3/1
  iu_sw/1 -> Out1/1
  thresh_sw/1 -> iw_sw/2, iv_sw/2, iu_sw/2
  Product/1 -> iv_sw/3
  const_iv/1 -> iv_sw/1
  Product2/1 -> iw_sw/3
  const_iw/1 -> iw_sw/1

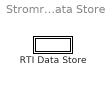
== system Stromregelkreis_old/RTI Data/RTI Data Store ==
  RTI Data Store : Subsystem  mask(RTI_DATA_STORE){}
      mask help:
      | RTI Data Store Block. This block is used by RTI to store internal model dependent data. Deleting this block will result in data loss.
      |
      | NEVER DELETE, COPY, OR MODIFY THIS BLOCK!
      mask Help:
      | RTI Data Store Block. This block is used by RTI to store internal model dependent data. Deleting this block will result in data loss.
      | 
      | NEVER DELETE, COPY, OR MODIFY THIS BLOCK!
      mask Display: text(0.5, 0.5, ' ', 'HorizontalAlignment', 'center');

== system Stromregelkreis_old/RTI Data/RTI Data Store/RTI Data Store ==
  RTI Data Store : Subsystem  mask(RTI_DATA_STORE){}
      mask help:
      | RTI Data Store Block. This block is used by RTI to store internal model dependent data. Deleting this block will result in data loss.
      |
      | NEVER DELETE, COPY, OR MODIFY THIS BLOCK!
      mask Help:
      | RTI Data Store Block. This block is used by RTI to store internal model dependent data. Deleting this block will result in data loss.
      | 
      | NEVER DELETE, COPY, OR MODIFY THIS BLOCK!
      mask Display: text(0.5, 0.5, ' ', 'HorizontalAlignment', 'center');

== system Stromregelkreis_old/RTI Data/RTI Data Store/RTI Data Store/RTI Data Store ==
  RTI Data Store : Subsystem  mask(RTI_DATA_STORE){}
      mask help:
      | RTI Data Store Block. This block is used by RTI to store internal model dependent data. Deleting this block will result in data loss.
      |
      | NEVER DELETE, COPY, OR MODIFY THIS BLOCK!
      mask Help:
      | RTI Data Store Block. This block is used by RTI to store internal model dependent data. Deleting this block will result in data loss.
      | 
      | NEVER DELETE, COPY, OR MODIFY THIS BLOCK!
      mask Display: text(0.5, 0.5, ' ', 'HorizontalAlignment', 'center');

== system Stromregelkreis_old/RTI Data/RTI Data Store/RTI Data Store/RTI Data Store/RTI Data Store ==
